simulink model "SSN_39busRT_Ctrl_4WT_19B"  (R2021a)
settings: Solver=ode3  StartTime=0.0  StopTime=10  FixedStep=Ts  MaxStep=1/60  RelTol=1e-2  AbsTol=1e-1
PreLoadFcn:
  | Ts=2.50e-6; ssn_ieee39_params; load('Pwf.mat');
InitFcn:
  | Ts=2.50e-6; ssn_ieee39_params; load('Pwf.mat');
values from neighbouring files (symbols this model uses):
  f = 50    [ssn_ieee39_params_ctrl.m]
  fNom = f    (= 60)    [ssn_ieee39_params_ctrl.m]
  ILR = 5.02    [ssn_ieee39_params_ctrl.m]
  IQMIN = 0.1    [ssn_ieee39_params_ctrl.m]
  ISCLIM = 1    [ssn_ieee39_params_ctrl.m]
  ITFpu = 1.10    (= 1.1)    [ssn_ieee39_params_ctrl.m]
  K = 1    [ssn_ieee39_params_ctrl.m]
  K1 = 1    [ssn_ieee39_params_ctrl.m]
  K2 = 2    [ssn_ieee39_params_ctrl.m]
  KCL = 1.04    [ssn_ieee39_params_ctrl.m]
  KFB = 0    [ssn_ieee39_params_ctrl.m]
  KFF = 1    [ssn_ieee39_params_ctrl.m]
  KFIX = 1    [ssn_ieee39_params_ctrl.m]
  KG = 1    [ssn_ieee39_params_ctrl.m]
  KIA = 59.91    [ssn_ieee39_params_ctrl.m]
  KIOEX = 0.0303    [ssn_ieee39_params_ctrl.m]
  KIUEX = 0.0303    [ssn_ieee39_params_ctrl.m]
  KIUOEX = 1    [ssn_ieee39_params_ctrl.m]
  KIUUEX = 1    [ssn_ieee39_params_ctrl.m]
  KLR = 22.47    [ssn_ieee39_params_ctrl.m]
  KM = 1    [ssn_ieee39_params_ctrl.m]
  KOEL = 0.24    [ssn_ieee39_params_ctrl.m]
  Kp = 1    [ssn_ieee39_params_ctrl.m]
  KPA = 30    [ssn_ieee39_params_ctrl.m]
  KPOEL = 1    [ssn_ieee39_params_ctrl.m]
  KPOEX = 0    [ssn_ieee39_params_ctrl.m]
  KPUEX = 0    [ssn_ieee39_params_ctrl.m]
  KSCALE = 0.319    [ssn_ieee39_params_ctrl.m]
  KUF = 0    [ssn_ieee39_params_ctrl.m]
  KUI = 0.001    [ssn_ieee39_params_ctrl.m]
  KUL = 0.24    [ssn_ieee39_params_ctrl.m]
  s = 10    [ssn_ieee39_params_ctrl.m]
  TA = 0.01    [ssn_ieee39_params_ctrl.m]
  Tadj = 0    [ssn_ieee39_params_ctrl.m]
  taps = [1 1 1.07 1.07 1.009 1.025 1 1.025 1.025 1.025]*1    [ssn_ieee39_params_ctrl.m]
  TF = 0.02    [ssn_ieee39_params_ctrl.m]
  TG = 0.024    [ssn_ieee39_params_ctrl.m]
  TINV = 0    [ssn_ieee39_params_ctrl.m]
  TIT = 0.1    [ssn_ieee39_params_ctrl.m]
  TL_10_11_len = 14    [ssn_ieee39_params_ctrl.m]
  TL_10_13_len = 14    [ssn_ieee39_params_ctrl.m]
  TL_13_14_len = 32    [ssn_ieee39_params_ctrl.m]
  TL_14_15_len = 70    [ssn_ieee39_params_ctrl.m]
  TL_15_16_len = 31.5    [ssn_ieee39_params_ctrl.m]
  TL_16_17_len = 26    [ssn_ieee39_params_ctrl.m]
  TL_16_19_len = 61    [ssn_ieee39_params_ctrl.m]
  TL_16_21_len = 46    [ssn_ieee39_params_ctrl.m]
  TL_16_24_len = 15    [ssn_ieee39_params_ctrl.m]
  TL_17_18_len = 26    [ssn_ieee39_params_ctrl.m]
  TL_17_27_len = 59    [ssn_ieee39_params_ctrl.m]
  TL_1_2_len = 134    [ssn_ieee39_params_ctrl.m]
  TL_1_39_len = 105    [ssn_ieee39_params_ctrl.m]
  TL_21_22_len = 47    [ssn_ieee39_params_ctrl.m]
  TL_22_23_len = 33    [ssn_ieee39_params_ctrl.m]
  TL_24_23_len = 88    [ssn_ieee39_params_ctrl.m]
  TL_25_26_len = 101    [ssn_ieee39_params_ctrl.m]
  TL_26_27_len = 46.5    [ssn_ieee39_params_ctrl.m]
  TL_26_28_len = 151    [ssn_ieee39_params_ctrl.m]
  TL_26_29_len = 200    [ssn_ieee39_params_ctrl.m]
  TL_28_29_len = 48    [ssn_ieee39_params_ctrl.m]
  TL_2_25_len = 28    [ssn_ieee39_params_ctrl.m]
  TL_2_2_len = 49    [ssn_ieee39_params_ctrl.m]
  TL_3_18_len = 42    [ssn_ieee39_params_ctrl.m]
  TL_3_4_len = 53    [ssn_ieee39_params_ctrl.m]
  TL_4_14_len = 33    [ssn_ieee39_params_ctrl.m]
  TL_4_5_len = 32.5    [ssn_ieee39_params_ctrl.m]
  TL_5_6_len = 14    [ssn_ieee39_params_ctrl.m]
  TL_5_8_len = 32    [ssn_ieee39_params_ctrl.m]
  TL_6_11_len = 26.5    [ssn_ieee39_params_ctrl.m]
  TL_6_7_len = 25.5    [ssn_ieee39_params_ctrl.m]
  TL_7_8_len = 15    [ssn_ieee39_params_ctrl.m]
  TL_8_9_len = 93    [ssn_ieee39_params_ctrl.m]
  TL_9_39_len = 136    [ssn_ieee39_params_ctrl.m]
  TOEL = 5.00    (= 5)    [ssn_ieee39_params_ctrl.m]
  TQREF = 0    [ssn_ieee39_params_ctrl.m]
  TQSCL = 0.012    [ssn_ieee39_params_ctrl.m]
  Ts_PMU = 1/1000    (= 0.001)    [ssn_ieee39_params_ctrl.m]
  TU1 = 0    [ssn_ieee39_params_ctrl.m]
  TU2 = 0    [ssn_ieee39_params_ctrl.m]
  TU3 = 0    [ssn_ieee39_params_ctrl.m]
  TU4 = 0    [ssn_ieee39_params_ctrl.m]
  TUL = 0    [ssn_ieee39_params_ctrl.m]
  TUP = 0.050    (= 0.05)    [ssn_ieee39_params_ctrl.m]
  TUQ = .005    (= 0.005)    [ssn_ieee39_params_ctrl.m]
  TUV = 0.2    [ssn_ieee39_params_ctrl.m]
  VAAMAX = VAMAX    (= 7.05)    [ssn_ieee39_params_ctrl.m]
  VAMAX = 7.05    [ssn_ieee39_params_ctrl.m]
  VAMIN = -6.11    [ssn_ieee39_params_ctrl.m]
  VBMAX = 999    [ssn_ieee39_params_ctrl.m]
  VF = 0    [ssn_ieee39_params_ctrl.m]
  VFB = 0    [ssn_ieee39_params_ctrl.m]
  VMMAX = 7.05    [ssn_ieee39_params_ctrl.m]
  VMMIN = -6.11    [ssn_ieee39_params_ctrl.m]
  VOELmax1 = 0.2353    [ssn_ieee39_params_ctrl.m]
  VOELmax2 = 0.0    (= 0)    [ssn_ieee39_params_ctrl.m]
  VOELmin1 = -0.24    [ssn_ieee39_params_ctrl.m]
  VOELmin2 = -1.0    (= -1)    [ssn_ieee39_params_ctrl.m]
  VRMAX = 7.05    [ssn_ieee39_params_ctrl.m]
  VRMIN = -6.11    [ssn_ieee39_params_ctrl.m]
  VSCLmax = 0.20    (= 0.2)    [ssn_ieee39_params_ctrl.m]
  VSCLmin = -0.10    (= -0.1)    [ssn_ieee39_params_ctrl.m]
  VUELmax1 = 1    [ssn_ieee39_params_ctrl.m]
  VUELmax2 = 1    [ssn_ieee39_params_ctrl.m]
  VUELmin1 = -1    [ssn_ieee39_params_ctrl.m]
  VUELmin2 = -1    [ssn_ieee39_params_ctrl.m]
  VUImax = 1    [ssn_ieee39_params_ctrl.m]
  VUImin = -1    [ssn_ieee39_params_ctrl.m]
undefined symbols (not defined in the file or in its folder): another_event_name, D1, Delta, DiscIntNeverNeededParam, find_system, MOV_segment9, my_event_name, powergui, Pw1, Pw2, Pw3, Pw4, vNomHV
libraries: powerlib_extras x162, spsThreePhaseVIMeasurementLib x55, spsCurrentMeasurementLib x52, simulink_extras x44, slpidlib x40, op_dpl_lib x36, spsST2AModel x20, spsThreePhaseParallelRLCLoadLib x20, spsThreePhaseTransformerTwoWindingsLib x17, spsControlledVoltageSourceLib x16, spsVoltageMeasurementLib x12, spsSynchronousMachinepuStandardLib x10
(part 5 of 19)

== system SSN_39busRT_Ctrl_4WT_19B/SM_master/G10/G10 ==
  note: Rotor Speed
  note: Rotor Speed Reference
  note: SM Measurement Signal
  note: Active Power
  note: Field Current
  note: Voltage Reference
  note: Stator Voltage
  note: Reactive Power
  note: Stator Current
  note: Field Voltage (Vf)
  note: Mechanical
      | Power (Pm)
  note: Measurement Outputs
  note: Rotor Speed
  note: Active Power
  note: Stator Voltage
  note: Stator Current
  note: Field Current
  note: Reactive Power
  wref (pu) : Inport
  Vref (pu) : Inport  Port=2
  "Generator Measurements " : Subsystem
  "Governor model " : Subsystem
  Ground7 : Ground
  ST6C EXCITER-1 : Subsystem
  Synchronous Machine : spsSynchronousMachinepuStandardLib/Synchronous Machine pu Standard  PresetModel=No  MechanicalLoad=Mechanical power Pm  ShowDetailedParameters=on  RotorType=Salient-pole  Units=per unit standard parameters  MeasurementBus=off  NominalParameters="[ Pn  Vn   f ]"  Reactances1=[ 31 32 33 34 35 36 37 ]  Reactances2=[ 1.305, 0.296, 0.252, 0.474, 0.243, 0.18 ]  dAxisTimeConstants=Short-circuit  qAxisTimeConstants=Open-circuit  TimeConstants1=[]  TimeConstants2=[]  TimeConstants3=[]  TimeConstants4=[]  TimeConstants5=[ 1.01, 0.053, 0.1 ]  TimeConstants6=[]  TimeConstants7=[]  TimeConstants8=[]  StatorResistance=2.8544e-3  Mechanical=[H1 0 2]  PolePairs=2  InitialConditions=[0 -62.5202 1.01055 1.01055 1.01055 8.25986 -111.74 128.26 1.32748]  SetSaturation=off  Saturation=[0.6404,0.7127,0.8441,0.9214,0.9956,1.082,1.19,1.316,1.457;0.7,0.7698,0.8872,0.9466,0.9969,1.046,1.1,1.151,1.201]  LoadFlowParameters=[1 150000000 0 0]  TsPowergui=0  TsBlock=-1  IterativeModel=Trapezoidal non iterative  IterativeDiscreteModel=Trapezoidal non iterative  BusType=PV  Pref=42e6  Qref=0  Qmin=-50000000  Qmax=50000000  PLF=0  QLF=0
      settings: SourceProductBaseCode=PS
  A : PMIOPort  Side=Right
  B : PMIOPort  Port=2  Side=Right
  C : PMIOPort  Port=3  Side=Right
  sm1 : Outport  VectorParamsAs1DForOutWhenUnconnected=off
  wires:
  [PT1st] -> "Governor model "/3(Input)
  [Ifd1st] -> ST6C EXCITER-1/4(Ifd)
  [Vt1st] -> ST6C EXCITER-1/2(Vt)
  [wm1] -> "Governor model "/2(w (pu))
  "Generator Measurements "/3(Vt) -> [Vt1st]
  "Generator Measurements "/6(PT) -> [PT1st]
  "Generator Measurements "/7(QT) -> [QT1st]
  "Generator Measurements "/1(sm) -> sm1/1
  "Generator Measurements "/5(It) -> [It1st]
  "Generator Measurements "/4(Ifd) -> [Ifd1st]
  "Generator Measurements "/2(wm) -> [wm1]
  ST6C EXCITER-1/1(Efd) -> Synchronous Machine/2, [Efd1st]
  [PT1st] -> ST6C EXCITER-1/7(PT)
  [It1st] -> ST6C EXCITER-1/3(It)
  [QT1st] -> ST6C EXCITER-1/6(QT)
  Ground7/1 -> ST6C EXCITER-1/5(Vstab)
  wref (pu)/1 -> "Governor model "/1(wref (pu)1)
  "Governor model "/1(Pmec (pu)) -> Synchronous Machine/1
  Vref (pu)/1 -> ST6C EXCITER-1/1(Vref)
  Synchronous Machine/1 -> "Generator Measurements "/1(m)
  connections:
  A/RConn1 -- Synchronous Machine/RConn1
  C/RConn1 -- Synchronous Machine/RConn3
  B/RConn1 -- Synchronous Machine/RConn2

== system SSN_39busRT_Ctrl_4WT_19B/SM_master/G2/G2 ==
  note: Reactive Power
  note: Field Current
  note: Stator Current
  note: Stator Voltage
  note: Active Power
  note: Rotor Speed
  note: Measurement Outputs
  note: Mechanical
      | Power (Pm)
  note: Field Voltage (Vf)
  note: Stator Current
  note: Reactive Power
  note: Stator Voltage
  note: Voltage Reference
  note: Field Current
  note: Active Power
  note: SM Measurement Signal
  note: Rotor Speed Reference
  note: Rotor Speed
  wref (pu) : Inport
  Vref (pu) : Inport  Port=2
  Generator Measurements (Output) : Subsystem
  "Governor model " : Subsystem
  Ground7 : Ground
  ST6C EXCITER-1 : Subsystem
  Synchronous Machine : spsSynchronousMachinepuStandardLib/Synchronous Machine pu Standard  PresetModel=No  MechanicalLoad=Mechanical power Pm  ShowDetailedParameters=on  RotorType=Salient-pole  Units=per unit standard parameters  MeasurementBus=off  NominalParameters="[ Pn  Vn   f ]"  Reactances1=[ 31 32 33 34 35 36 37 ]  Reactances2=[ 1.305, 0.296, 0.252, 0.474, 0.243, 0.18 ]  dAxisTimeConstants=Short-circuit  qAxisTimeConstants=Open-circuit  TimeConstants1=[]  TimeConstants2=[]  TimeConstants3=[]  TimeConstants4=[]  TimeConstants5=[ 1.01, 0.053, 0.1 ]  TimeConstants6=[]  TimeConstants7=[]  TimeConstants8=[]  StatorResistance=2.8544e-3  Mechanical=[H1 0 2]  PolePairs=2  InitialConditions=[0 -62.5202 1.01055 1.01055 1.01055 8.25986 -111.74 128.26 1.32748]  SetSaturation=off  Saturation=[0.6404,0.7127,0.8441,0.9214,0.9956,1.082,1.19,1.316,1.457;0.7,0.7698,0.8872,0.9466,0.9969,1.046,1.1,1.151,1.201]  LoadFlowParameters=[1 150000000 0 0]  TsPowergui=0  TsBlock=-1  IterativeModel=Trapezoidal non iterative  IterativeDiscreteModel=Trapezoidal non iterative  BusType=PV  Pref=42e6  Qref=0  Qmin=-50000000  Qmax=50000000  PLF=0  QLF=0
      settings: SourceProductBaseCode=PS
  A : PMIOPort  Side=Right
  B : PMIOPort  Port=2  Side=Right
  C : PMIOPort  Port=3  Side=Right
  sm1 : Outport  VectorParamsAs1DForOutWhenUnconnected=off
  wires:
  Synchronous Machine/1 -> Generator Measurements (Output)/1(m)
  Vref (pu)/1 -> ST6C EXCITER-1/1(Vref)
  "Governor model "/1(Pmec (pu)) -> Synchronous Machine/1
  wref (pu)/1 -> "Governor model "/1(wref (pu)1)
  Ground7/1 -> ST6C EXCITER-1/5(Vstab)
  [QT1st] -> ST6C EXCITER-1/6(QT)
  [It1st] -> ST6C EXCITER-1/3(It)
  [PT1st] -> ST6C EXCITER-1/7(PT)
  ST6C EXCITER-1/1(Efd) -> [Efd1st], Synchronous Machine/2
  Generator Measurements (Output)/2(wm) -> [wm1]
  Generator Measurements (Output)/4(Ifd) -> [Ifd1st]
  Generator Measurements (Output)/5(It) -> [It1st]
  Generator Measurements (Output)/1(sm) -> sm1/1
  Generator Measurements (Output)/7(QT) -> [QT1st]
  Generator Measurements (Output)/6(PT) -> [PT1st]
  Generator Measurements (Output)/3(Vt) -> [Vt1st]
  [wm1] -> "Governor model "/2(w (pu))
  [Vt1st] -> ST6C EXCITER-1/2(Vt)
  [Ifd1st] -> ST6C EXCITER-1/4(Ifd)
  [PT1st] -> "Governor model "/3(Input)
  connections:
  B/RConn1 -- Synchronous Machine/RConn2
  C/RConn1 -- Synchronous Machine/RConn3
  A/RConn1 -- Synchronous Machine/RConn1

== system SSN_39busRT_Ctrl_4WT_19B/SM_master/G3/G3 ==
  note: Rotor Speed
  note: Rotor Speed Reference
  note: SM Measurement Signal
  note: Active Power
  note: Field Current
  note: Voltage Reference
  note: Stator Voltage
  note: Reactive Power
  note: Stator Current
  note: Field Voltage (Vf)
  note: Synchronous
      | Machine
      | - Phase A
      | - Phase B
      | - Phase C
  note: Mechanical
      | Power (Pm)
  note: Selected (Combined)
      | Synchronous Machine
      | Measurement Outputs
  note: Rotor Speed
  note: Active Power
  note: Stator Voltage
  note: Stator Current
  note: Field Current
  note: Reactive Power
  wref (pu) : Inport
  Vref (pu) : Inport  Port=2
  Generator Measurements (Output) : Subsystem
  Governor model with Droop : Subsystem
  Ground7 : Ground
  ST6C EXCITER-1 : Subsystem
  Synchronous Machine : spsSynchronousMachinepuStandardLib/Synchronous Machine pu Standard  PresetModel=No  MechanicalLoad=Mechanical power Pm  ShowDetailedParameters=on  RotorType=Salient-pole  Units=per unit standard parameters  MeasurementBus=off  NominalParameters="[ Pn  Vn   f ]"  Reactances1=[ 31 32 33 34 35 36 37 ]  Reactances2=[ 1.305, 0.296, 0.252, 0.474, 0.243, 0.18 ]  dAxisTimeConstants=Short-circuit  qAxisTimeConstants=Open-circuit  TimeConstants1=[]  TimeConstants2=[]  TimeConstants3=[]  TimeConstants4=[]  TimeConstants5=[ 1.01, 0.053, 0.1 ]  TimeConstants6=[]  TimeConstants7=[]  TimeConstants8=[]  StatorResistance=2.8544e-3  Mechanical=[H1 0 2]  PolePairs=2  InitialConditions=[0 -62.5202 1.01055 1.01055 1.01055 8.25986 -111.74 128.26 1.32748]  SetSaturation=off  Saturation=[0.6404,0.7127,0.8441,0.9214,0.9956,1.082,1.19,1.316,1.457;0.7,0.7698,0.8872,0.9466,0.9969,1.046,1.1,1.151,1.201]  LoadFlowParameters=[1 150000000 0 0]  TsPowergui=0  TsBlock=-1  IterativeModel=Trapezoidal non iterative  IterativeDiscreteModel=Trapezoidal non iterative  BusType=PV  Pref=42e6  Qref=0  Qmin=-50000000  Qmax=50000000  PLF=0  QLF=0
      settings: SourceProductBaseCode=PS
  A : PMIOPort  Side=Right
  B : PMIOPort  Port=2  Side=Right
  C : PMIOPort  Port=3  Side=Right
  sm1 : Outport  VectorParamsAs1DForOutWhenUnconnected=off
  wires:
  [PT1st] -> Governor model with Droop/3(Input)
  [Ifd1st] -> ST6C EXCITER-1/4(Ifd)
  [Vt1st] -> ST6C EXCITER-1/2(Vt)
  [wm1] -> Governor model with Droop/2(w (pu))
  Generator Measurements (Output)/3(Vt) -> [Vt1st]
  Generator Measurements (Output)/6(PT) -> [PT1st]
  Generator Measurements (Output)/7(QT) -> [QT1st]
  Generator Measurements (Output)/1(sm) -> sm1/1
  Generator Measurements (Output)/5(It) -> [It1st]
  Generator Measurements (Output)/4(Ifd) -> [Ifd1st]
  Generator Measurements (Output)/2(wm) -> [wm1]
  ST6C EXCITER-1/1(Efd) -> Synchronous Machine/2, [Efd1st]
  [PT1st] -> ST6C EXCITER-1/7(PT)
  [It1st] -> ST6C EXCITER-1/3(It)
  [QT1st] -> ST6C EXCITER-1/6(QT)
  Ground7/1 -> ST6C EXCITER-1/5(Vstab)
  wref (pu)/1 -> Governor model with Droop/1(wref (pu)1)
  Governor model with Droop/1(Pmec (pu)) -> Synchronous Machine/1
  Vref (pu)/1 -> ST6C EXCITER-1/1(Vref)
  Synchronous Machine/1 -> Generator Measurements (Output)/1(m)
  connections:
  A/RConn1 -- Synchronous Machine/RConn1
  C/RConn1 -- Synchronous Machine/RConn3
  B/RConn1 -- Synchronous Machine/RConn2

== system SSN_39busRT_Ctrl_4WT_19B/SM_master/G4/G4 ==
  note: Rotor Speed
  note: Rotor Speed Reference
  note: SM Measurement Signal
  note: Active Power
  note: Field Current
  note: Voltage Reference
  note: Stator Voltage
  note: Reactive Power
  note: Stator Current
  note: Field Voltage (Vf)
  note: Mechanical
      | Power (Pm)
  note: Measurement Outputs
  note: Rotor Speed
  note: Active Power
  note: Stator Voltage
  note: Stator Current
  note: Field Current
  note: Reactive Power
  wref (pu) : Inport
  Vref (pu) : Inport  Port=2
  Generator Measurements (Output) : Subsystem
  "Governor model " : Subsystem
  Ground7 : Ground
  ST6C EXCITER-1 : Subsystem
  Synchronous Machine : spsSynchronousMachinepuStandardLib/Synchronous Machine pu Standard  PresetModel=No  MechanicalLoad=Mechanical power Pm  ShowDetailedParameters=on  RotorType=Salient-pole  Units=per unit standard parameters  MeasurementBus=off  NominalParameters="[ Pn  Vn   f ]"  Reactances1=[ 31 32 33 34 35 36 37 ]  Reactances2=[ 1.305, 0.296, 0.252, 0.474, 0.243, 0.18 ]  dAxisTimeConstants=Short-circuit  qAxisTimeConstants=Open-circuit  TimeConstants1=[]  TimeConstants2=[]  TimeConstants3=[]  TimeConstants4=[]  TimeConstants5=[ 1.01, 0.053, 0.1 ]  TimeConstants6=[]  TimeConstants7=[]  TimeConstants8=[]  StatorResistance=2.8544e-3  Mechanical=[H1 0 2]  PolePairs=2  InitialConditions=[0 -62.5202 1.01055 1.01055 1.01055 8.25986 -111.74 128.26 1.32748]  SetSaturation=off  Saturation=[0.6404,0.7127,0.8441,0.9214,0.9956,1.082,1.19,1.316,1.457;0.7,0.7698,0.8872,0.9466,0.9969,1.046,1.1,1.151,1.201]  LoadFlowParameters=[1 150000000 0 0]  TsPowergui=0  TsBlock=-1  IterativeModel=Trapezoidal non iterative  IterativeDiscreteModel=Trapezoidal non iterative  BusType=PV  Pref=42e6  Qref=0  Qmin=-50000000  Qmax=50000000  PLF=0  QLF=0
      settings: SourceProductBaseCode=PS
  A : PMIOPort  Side=Right
  B : PMIOPort  Port=2  Side=Right
  C : PMIOPort  Port=3  Side=Right
  sm1 : Outport  VectorParamsAs1DForOutWhenUnconnected=off
  wires:
  [PT1st] -> "Governor model "/3(Input)
  [Ifd1st] -> ST6C EXCITER-1/4(Ifd)
  [Vt1st] -> ST6C EXCITER-1/2(Vt)
  [wm1] -> "Governor model "/2(w (pu))
  Generator Measurements (Output)/3(Vt) -> [Vt1st]
  Generator Measurements (Output)/6(PT) -> [PT1st]
  Generator Measurements (Output)/7(QT) -> [QT1st]
  Generator Measurements (Output)/1(sm) -> sm1/1
  Generator Measurements (Output)/5(It) -> [It1st]
  Generator Measurements (Output)/4(Ifd) -> [Ifd1st]
  Generator Measurements (Output)/2(wm) -> [wm1]
  ST6C EXCITER-1/1(Efd) -> Synchronous Machine/2, [Efd1st]
  [PT1st] -> ST6C EXCITER-1/7(PT)
  [It1st] -> ST6C EXCITER-1/3(It)
  [QT1st] -> ST6C EXCITER-1/6(QT)
  Ground7/1 -> ST6C EXCITER-1/5(Vstab)
  wref (pu)/1 -> "Governor model "/1(wref (pu)1)
  "Governor model "/1(Pmec (pu)) -> Synchronous Machine/1
  Vref (pu)/1 -> ST6C EXCITER-1/1(Vref)
  Synchronous Machine/1 -> Generator Measurements (Output)/1(m)
  connections:
  A/RConn1 -- Synchronous Machine/RConn1
  C/RConn1 -- Synchronous Machine/RConn3
  B/RConn1 -- Synchronous Machine/RConn2

== system SSN_39busRT_Ctrl_4WT_19B/SM_master/G5/G5 ==
  note: Reactive Power
  note: Field Current
  note: Stator Current
  note: Stator Voltage
  note: Active Power
  note: Rotor Speed
  note: Selected (Combined)
      | Synchronous Machine
      | Measurement Outputs
  note: Mechanical
      | Power (Pm)
  note: Synchronous
      | Machine
      | - Phase A
      | - Phase B
      | - Phase C
  note: Field Voltage (Vf)
  note: Stator Current
  note: Reactive Power
  note: Stator Voltage
  note: Voltage Reference
  note: Field Current
  note: Active Power
  note: SM Measurement Signal
  note: Rotor Speed Reference
  note: Rotor Speed
  wref (pu) : Inport
  Vref (pu) : Inport  Port=2
  Generator Measurements (Output) : Subsystem
  Governor model with Droop : Subsystem
  Ground7 : Ground
  ST6C EXCITER-1 : Subsystem
  Synchronous Machine : spsSynchronousMachinepuStandardLib/Synchronous Machine pu Standard  PresetModel=No  MechanicalLoad=Mechanical power Pm  ShowDetailedParameters=on  RotorType=Salient-pole  Units=per unit standard parameters  MeasurementBus=off  NominalParameters="[ Pn  Vn   f ]"  Reactances1=[ 31 32 33 34 35 36 37 ]  Reactances2=[ 1.305, 0.296, 0.252, 0.474, 0.243, 0.18 ]  dAxisTimeConstants=Short-circuit  qAxisTimeConstants=Open-circuit  TimeConstants1=[]  TimeConstants2=[]  TimeConstants3=[]  TimeConstants4=[]  TimeConstants5=[ 1.01, 0.053, 0.1 ]  TimeConstants6=[]  TimeConstants7=[]  TimeConstants8=[]  StatorResistance=2.8544e-3  Mechanical=[H1 0 2]  PolePairs=2  InitialConditions=[0 -62.5202 1.01055 1.01055 1.01055 8.25986 -111.74 128.26 1.32748]  SetSaturation=off  Saturation=[0.6404,0.7127,0.8441,0.9214,0.9956,1.082,1.19,1.316,1.457;0.7,0.7698,0.8872,0.9466,0.9969,1.046,1.1,1.151,1.201]  LoadFlowParameters=[1 150000000 0 0]  TsPowergui=0  TsBlock=-1  IterativeModel=Trapezoidal non iterative  IterativeDiscreteModel=Trapezoidal non iterative  BusType=PV  Pref=42e6  Qref=0  Qmin=-50000000  Qmax=50000000  PLF=0  QLF=0
      settings: SourceProductBaseCode=PS
  A : PMIOPort  Side=Right
  B : PMIOPort  Port=2  Side=Right
  C : PMIOPort  Port=3  Side=Right
  sm1 : Outport  VectorParamsAs1DForOutWhenUnconnected=off
  wires:
  Synchronous Machine/1 -> Generator Measurements (Output)/1(m)
  Vref (pu)/1 -> ST6C EXCITER-1/1(Vref)
  Governor model with Droop/1(Pmec (pu)) -> Synchronous Machine/1
  wref (pu)/1 -> Governor model with Droop/1(wref (pu)1)
  Ground7/1 -> ST6C EXCITER-1/5(Vstab)
  [QT1st] -> ST6C EXCITER-1/6(QT)
  [It1st] -> ST6C EXCITER-1/3(It)
  [PT1st] -> ST6C EXCITER-1/7(PT)
  ST6C EXCITER-1/1(Efd) -> [Efd1st], Synchronous Machine/2
  Generator Measurements (Output)/2(wm) -> [wm1]
  Generator Measurements (Output)/4(Ifd) -> [Ifd1st]
  Generator Measurements (Output)/5(It) -> [It1st]
  Generator Measurements (Output)/1(sm) -> sm1/1
  Generator Measurements (Output)/7(QT) -> [QT1st]
  Generator Measurements (Output)/6(PT) -> [PT1st]
  Generator Measurements (Output)/3(Vt) -> [Vt1st]
  [wm1] -> Governor model with Droop/2(w (pu))
  [Vt1st] -> ST6C EXCITER-1/2(Vt)
  [Ifd1st] -> ST6C EXCITER-1/4(Ifd)
  [PT1st] -> Governor model with Droop/3(Input)
  connections:
  B/RConn1 -- Synchronous Machine/RConn2
  C/RConn1 -- Synchronous Machine/RConn3
  A/RConn1 -- Synchronous Machine/RConn1

== system SSN_39busRT_Ctrl_4WT_19B/SM_master/G6/G6 ==
  note: Rotor Speed
  note: Rotor Speed Reference
  note: SM Measurement Signal
  note: Active Power
  note: Field Current
  note: Voltage Reference
  note: Stator Voltage
  note: Reactive Power
  note: Stator Current
  note: Field Voltage (Vf)
  note: Mechanical
      | Power (Pm)
  note: Measurement Outputs
  note: Rotor Speed
  note: Active Power
  note: Stator Voltage
  note: Stator Current
  note: Field Current
  note: Reactive Power
  wref (pu) : Inport
  Vref (pu) : Inport  Port=2
  Generator Measurements (Output) : Subsystem
  Governor model with Droop : Subsystem
  Ground7 : Ground
  ST6C EXCITER-1 : Subsystem
  Synchronous Machine : spsSynchronousMachinepuStandardLib/Synchronous Machine pu Standard  PresetModel=No  MechanicalLoad=Mechanical power Pm  ShowDetailedParameters=on  RotorType=Salient-pole  Units=per unit standard parameters  MeasurementBus=off  NominalParameters="[ Pn  Vn   f ]"  Reactances1=[ 31 32 33 34 35 36 37 ]  Reactances2=[ 1.305, 0.296, 0.252, 0.474, 0.243, 0.18 ]  dAxisTimeConstants=Short-circuit  qAxisTimeConstants=Open-circuit  TimeConstants1=[]  TimeConstants2=[]  TimeConstants3=[]  TimeConstants4=[]  TimeConstants5=[ 1.01, 0.053, 0.1 ]  TimeConstants6=[]  TimeConstants7=[]  TimeConstants8=[]  StatorResistance=2.8544e-3  Mechanical=[H1 0 2]  PolePairs=2  InitialConditions=[0 -62.5202 1.01055 1.01055 1.01055 8.25986 -111.74 128.26 1.32748]  SetSaturation=off  Saturation=[0.6404,0.7127,0.8441,0.9214,0.9956,1.082,1.19,1.316,1.457;0.7,0.7698,0.8872,0.9466,0.9969,1.046,1.1,1.151,1.201]  LoadFlowParameters=[1 150000000 0 0]  TsPowergui=0  TsBlock=-1  IterativeModel=Trapezoidal non iterative  IterativeDiscreteModel=Trapezoidal non iterative  BusType=PV  Pref=42e6  Qref=0  Qmin=-50000000  Qmax=50000000  PLF=0  QLF=0
      settings: SourceProductBaseCode=PS
  A : PMIOPort  Side=Right
  B : PMIOPort  Port=2  Side=Right
  C : PMIOPort  Port=3  Side=Right
  sm1 : Outport  VectorParamsAs1DForOutWhenUnconnected=off
  wires:
  [PT1st] -> Governor model with Droop/3(Input)
  [Ifd1st] -> ST6C EXCITER-1/4(Ifd)
  [Vt1st] -> ST6C EXCITER-1/2(Vt)
  [wm1] -> Governor model with Droop/2(w (pu))
  Generator Measurements (Output)/3(Vt) -> [Vt1st]
  Generator Measurements (Output)/6(PT) -> [PT1st]
  Generator Measurements (Output)/7(QT) -> [QT1st]
  Generator Measurements (Output)/1(sm) -> sm1/1
  Generator Measurements (Output)/5(It) -> [It1st]
  Generator Measurements (Output)/4(Ifd) -> [Ifd1st]
  Generator Measurements (Output)/2(wm) -> [wm1]
  ST6C EXCITER-1/1(Efd) -> Synchronous Machine/2, [Efd1st]
  [PT1st] -> ST6C EXCITER-1/7(PT)
  [It1st] -> ST6C EXCITER-1/3(It)
  [QT1st] -> ST6C EXCITER-1/6(QT)
  Ground7/1 -> ST6C EXCITER-1/5(Vstab)
  wref (pu)/1 -> Governor model with Droop/1(wref (pu)1)
  Governor model with Droop/1(Pmec (pu)) -> Synchronous Machine/1
  Vref (pu)/1 -> ST6C EXCITER-1/1(Vref)
  Synchronous Machine/1 -> Generator Measurements (Output)/1(m)
  connections:
  A/RConn1 -- Synchronous Machine/RConn1
  C/RConn1 -- Synchronous Machine/RConn3
  B/RConn1 -- Synchronous Machine/RConn2

== system SSN_39busRT_Ctrl_4WT_19B/SM_master/G7/G7 ==
  note: Rotor Speed
  note: Rotor Speed Reference
  note: SM Measurement Signal
  note: Active Power
  note: Field Current
  note: Voltage Reference
  note: Stator Voltage
  note: Reactive Power
  note: Stator Current
  note: Field Voltage (Vf)
  note: Mechanical
      | Power (Pm)
  note: Measurement Outputs
  note: Rotor Speed
  note: Active Power
  note: Stator Voltage
  note: Stator Current
  note: Field Current
  note: Reactive Power
  wref (pu) : Inport
  Vref (pu) : Inport  Port=2
  Generator Measurements (Output) : Subsystem
  Governor model with Droop : Subsystem
  Ground7 : Ground
  ST6C EXCITER-1 : Subsystem
  Synchronous Machine : spsSynchronousMachinepuStandardLib/Synchronous Machine pu Standard  PresetModel=No  MechanicalLoad=Mechanical power Pm  ShowDetailedParameters=on  RotorType=Salient-pole  Units=per unit standard parameters  MeasurementBus=off  NominalParameters="[ Pn  Vn   f ]"  Reactances1=[ 31 32 33 34 35 36 37 ]  Reactances2=[ 1.305, 0.296, 0.252, 0.474, 0.243, 0.18 ]  dAxisTimeConstants=Short-circuit  qAxisTimeConstants=Open-circuit  TimeConstants1=[]  TimeConstants2=[]  TimeConstants3=[]  TimeConstants4=[]  TimeConstants5=[ 1.01, 0.053, 0.1 ]  TimeConstants6=[]  TimeConstants7=[]  TimeConstants8=[]  StatorResistance=2.8544e-3  Mechanical=[H1 0 2]  PolePairs=2  InitialConditions=[0 -62.5202 1.01055 1.01055 1.01055 8.25986 -111.74 128.26 1.32748]  SetSaturation=off  Saturation=[0.6404,0.7127,0.8441,0.9214,0.9956,1.082,1.19,1.316,1.457;0.7,0.7698,0.8872,0.9466,0.9969,1.046,1.1,1.151,1.201]  LoadFlowParameters=[1 150000000 0 0]  TsPowergui=0  TsBlock=-1  IterativeModel=Trapezoidal non iterative  IterativeDiscreteModel=Trapezoidal non iterative  BusType=PV  Pref=42e6  Qref=0  Qmin=-50000000  Qmax=50000000  PLF=0  QLF=0
      settings: SourceProductBaseCode=PS
  A : PMIOPort  Side=Right
  B : PMIOPort  Port=2  Side=Right
  C : PMIOPort  Port=3  Side=Right
  sm1 : Outport  VectorParamsAs1DForOutWhenUnconnected=off
  wires:
  [PT1st] -> Governor model with Droop/3(Input)
  [Ifd1st] -> ST6C EXCITER-1/4(Ifd)
  [Vt1st] -> ST6C EXCITER-1/2(Vt)
  [wm1] -> Governor model with Droop/2(w (pu))
  Generator Measurements (Output)/3(Vt) -> [Vt1st]
  Generator Measurements (Output)/6(PT) -> [PT1st]
  Generator Measurements (Output)/7(QT) -> [QT1st]
  Generator Measurements (Output)/1(sm) -> sm1/1
  Generator Measurements (Output)/5(It) -> [It1st]
  Generator Measurements (Output)/4(Ifd) -> [Ifd1st]
  Generator Measurements (Output)/2(wm) -> [wm1]
  ST6C EXCITER-1/1(Efd) -> Synchronous Machine/2, [Efd1st]
  [PT1st] -> ST6C EXCITER-1/7(PT)
  [It1st] -> ST6C EXCITER-1/3(It)
  [QT1st] -> ST6C EXCITER-1/6(QT)
  Ground7/1 -> ST6C EXCITER-1/5(Vstab)
  wref (pu)/1 -> Governor model with Droop/1(wref (pu)1)
  Governor model with Droop/1(Pmec (pu)) -> Synchronous Machine/1
  Vref (pu)/1 -> ST6C EXCITER-1/1(Vref)
  Synchronous Machine/1 -> Generator Measurements (Output)/1(m)
  connections:
  A/RConn1 -- Synchronous Machine/RConn1
  C/RConn1 -- Synchronous Machine/RConn3
  B/RConn1 -- Synchronous Machine/RConn2

== system SSN_39busRT_Ctrl_4WT_19B/SM_master/G8/ G8 ==
  note: Reactive Power
  note: Field Current
  note: Stator Current
  note: Stator Voltage
  note: Active Power
  note: Rotor Speed
  note: Measurement Outputs
  note: Mechanical
      | Power (PU)
  note: Field Voltage (Vf PU)
  note: Stator Current
  note: Reactive Power
  note: Stator Voltage
  note: Voltage Reference
  note: Field Current
  note: Active Power
  note: SM Measurement Signal
  note: Rotor Speed Reference
  note: Rotor Speed
  wref (pu) : Inport
  Vref (pu) : Inport  Port=2
  "Generator Measurements " : Subsystem
  "Governor model " : Subsystem
  Ground7 : Ground
  ST6C EXCITER-1 : Subsystem
  Synchronous Machine : spsSynchronousMachinepuStandardLib/Synchronous Machine pu Standard  PresetModel=No  MechanicalLoad=Mechanical power Pm  ShowDetailedParameters=on  RotorType=Salient-pole  Units=per unit standard parameters  MeasurementBus=off  NominalParameters="[ Pn  Vn   f ]"  Reactances1=[ 31 32 33 34 35 36 37 ]  Reactances2=[ 1.305, 0.296, 0.252, 0.474, 0.243, 0.18 ]  dAxisTimeConstants=Short-circuit  qAxisTimeConstants=Open-circuit  TimeConstants1=[]  TimeConstants2=[]  TimeConstants3=[]  TimeConstants4=[]  TimeConstants5=[ 1.01, 0.053, 0.1 ]  TimeConstants6=[]  TimeConstants7=[]  TimeConstants8=[]  StatorResistance=2.8544e-3  Mechanical=[H1 0 2]  PolePairs=2  InitialConditions=[0 -62.5202 1.01055 1.01055 1.01055 8.25986 -111.74 128.26 1.32748]  SetSaturation=off  Saturation=[0.6404,0.7127,0.8441,0.9214,0.9956,1.082,1.19,1.316,1.457;0.7,0.7698,0.8872,0.9466,0.9969,1.046,1.1,1.151,1.201]  LoadFlowParameters=[1 150000000 0 0]  TsPowergui=0  TsBlock=-1  IterativeModel=Trapezoidal non iterative  IterativeDiscreteModel=Trapezoidal non iterative  BusType=PV  Pref=42e6  Qref=0  Qmin=-50000000  Qmax=50000000  PLF=0  QLF=0
      settings: SourceProductBaseCode=PS
  A : PMIOPort  Side=Right
  B : PMIOPort  Port=2  Side=Right
  C : PMIOPort  Port=3  Side=Right
  sm1 : Outport  VectorParamsAs1DForOutWhenUnconnected=off
  wires:
  Synchronous Machine/1 -> "Generator Measurements "/1(m)
  Vref (pu)/1 -> ST6C EXCITER-1/1(Vref)
  "Governor model "/1(Pmec (pu)) -> Synchronous Machine/1
  wref (pu)/1 -> "Governor model "/1(wref (pu)1)
  Ground7/1 -> ST6C EXCITER-1/5(Vstab)
  [QT1st] -> ST6C EXCITER-1/6(QT)
  [It1st] -> ST6C EXCITER-1/3(It)
  [PT1st] -> ST6C EXCITER-1/7(PT)
  ST6C EXCITER-1/1(Efd) -> [Efd1st], Synchronous Machine/2
  "Generator Measurements "/2(wm) -> [wm1]
  "Generator Measurements "/4(Ifd) -> [Ifd1st]
  "Generator Measurements "/5(It) -> [It1st]
  "Generator Measurements "/1(sm) -> sm1/1
  "Generator Measurements "/7(QT) -> [QT1st]
  "Generator Measurements "/6(PT) -> [PT1st]
  "Generator Measurements "/3(Vt) -> [Vt1st]
  [wm1] -> "Governor model "/2(w (pu))
  [Vt1st] -> ST6C EXCITER-1/2(Vt)
  [Ifd1st] -> ST6C EXCITER-1/4(Ifd)
  [PT1st] -> "Governor model "/3(Input)
  connections:
  B/RConn1 -- Synchronous Machine/RConn2
  C/RConn1 -- Synchronous Machine/RConn3
  A/RConn1 -- Synchronous Machine/RConn1

== system SSN_39busRT_Ctrl_4WT_19B/SM_master/G9/G9 ==
  note: Rotor Speed
  note: Rotor Speed Reference
  note: SM Measurement Signal
  note: Active Power
  note: Field Current
  note: Voltage Reference
  note: Stator Voltage
  note: Reactive Power
  note: Stator Current
  note: Field Voltage (Vf)
  note: Mechanical
      | Power (Pm)
  note: Measurement Outputs
  note: Rotor Speed
  note: Active Power
  note: Stator Voltage
  note: Stator Current
  note: Field Current
  note: Reactive Power
  wref (pu) : Inport
  Vref (pu) : Inport  Port=2
  Generator Measurements (Output) : Subsystem
  Governor model with Droop : Subsystem
  Ground7 : Ground
  ST6C EXCITER-1 : Subsystem
  Synchronous Machine : spsSynchronousMachinepuStandardLib/Synchronous Machine pu Standard  PresetModel=No  MechanicalLoad=Mechanical power Pm  ShowDetailedParameters=on  RotorType=Salient-pole  Units=per unit standard parameters  MeasurementBus=off  NominalParameters="[ Pn  Vn   f ]"  Reactances1=[ 31 32 33 34 35 36 37 ]  Reactances2=[ 1.305, 0.296, 0.252, 0.474, 0.243, 0.18 ]  dAxisTimeConstants=Short-circuit  qAxisTimeConstants=Open-circuit  TimeConstants1=[]  TimeConstants2=[]  TimeConstants3=[]  TimeConstants4=[]  TimeConstants5=[ 1.01, 0.053, 0.1 ]  TimeConstants6=[]  TimeConstants7=[]  TimeConstants8=[]  StatorResistance=2.8544e-3  Mechanical=[H1 0 2]  PolePairs=2  InitialConditions=[0 -62.5202 1.01055 1.01055 1.01055 8.25986 -111.74 128.26 1.32748]  SetSaturation=off  Saturation=[0.6404,0.7127,0.8441,0.9214,0.9956,1.082,1.19,1.316,1.457;0.7,0.7698,0.8872,0.9466,0.9969,1.046,1.1,1.151,1.201]  LoadFlowParameters=[1 150000000 0 0]  TsPowergui=0  TsBlock=-1  IterativeModel=Trapezoidal non iterative  IterativeDiscreteModel=Trapezoidal non iterative  BusType=PV  Pref=42e6  Qref=0  Qmin=-50000000  Qmax=50000000  PLF=0  QLF=0
      settings: SourceProductBaseCode=PS
  A : PMIOPort  Side=Right
  B : PMIOPort  Port=2  Side=Right
  C : PMIOPort  Port=3  Side=Right
  sm1 : Outport  VectorParamsAs1DForOutWhenUnconnected=off
  wires:
  [PT1st] -> Governor model with Droop/3(Input)
  [Ifd1st] -> ST6C EXCITER-1/4(Ifd)
  [Vt1st] -> ST6C EXCITER-1/2(Vt)
  [wm1] -> Governor model with Droop/2(w (pu))
  Generator Measurements (Output)/3(Vt) -> [Vt1st]
  Generator Measurements (Output)/6(PT) -> [PT1st]
  Generator Measurements (Output)/7(QT) -> [QT1st]
  Generator Measurements (Output)/1(sm) -> sm1/1
  Generator Measurements (Output)/5(It) -> [It1st]
  Generator Measurements (Output)/4(Ifd) -> [Ifd1st]
  Generator Measurements (Output)/2(wm) -> [wm1]
  ST6C EXCITER-1/1(Efd) -> Synchronous Machine/2, [Efd1st]
  [PT1st] -> ST6C EXCITER-1/7(PT)
  [It1st] -> ST6C EXCITER-1/3(It)
  [QT1st] -> ST6C EXCITER-1/6(QT)
  Ground7/1 -> ST6C EXCITER-1/5(Vstab)
  wref (pu)/1 -> Governor model with Droop/1(wref (pu)1)
  Governor model with Droop/1(Pmec (pu)) -> Synchronous Machine/1
  Vref (pu)/1 -> ST6C EXCITER-1/1(Vref)
  Synchronous Machine/1 -> Generator Measurements (Output)/1(m)
  connections:
  A/RConn1 -- Synchronous Machine/RConn1
  C/RConn1 -- Synchronous Machine/RConn3
  B/RConn1 -- Synchronous Machine/RConn2

== system SSN_39busRT_Ctrl_4WT_19B/powergui/EquivalentModel1/Sources ==
  Mux : Mux  Inputs=[1 1]
  u : Outport  VectorParamsAs1DForOutWhenUnconnected=off
  wires:
  Mux/1 -> u/1
  [T159_13809_39445529444035] -> Mux/1
  [T160_13858_39325123805635] -> Mux/2

== system SSN_39busRT_Ctrl_4WT_19B/powergui/EquivalentModel1/Yout ==
  v,i : Inport
  Demux : Demux  Outputs=[1 1 1]
  tag scope: T149_12942_36324237428855=global, T166_14587_45637003886935=global, T167_14636_45637984399065=global
  wires:
  v,i/1 -> Demux/1
  Demux/1 -> [T166_14587_45637003886935]
  Demux/2 -> [T167_14636_45637984399065]
  Demux/3 -> [T149_12942_36324237428855]

== system SSN_39busRT_Ctrl_4WT_19B/powergui/EquivalentModel10/Sources ==
  Mux : Mux  Inputs=[2 1 1 1 1 1 1 1 1 1 1 1 1]
  u : Outport  VectorParamsAs1DForOutWhenUnconnected=off
  wires:
  Mux/1 -> u/1
  [T67_5835_7808160989715] -> Mux/1
  [T74_6142_7947224238180] -> Mux/2
  [T74_6143_7948232813167] -> Mux/3
  [T74_6144_7949457397884] -> Mux/4
  [T75_6197_8147459697777] -> Mux/5
  [T75_6198_8148543724566] -> Mux/6
  [T75_6199_8149847124422] -> Mux/7
  [T74_6144_7943290167466] -> Mux/8
  [T74_6145_7944295233974] -> Mux/9
  [T74_6146_7945516310213] -> Mux/10
  [T75_6194_8151564869885] -> Mux/11
  [T75_6195_8152655070811] -> Mux/12
  [T75_6196_8153964644804] -> Mux/13

== system SSN_39busRT_Ctrl_4WT_19B/powergui/EquivalentModel10/Yout ==
  v,i : Inport
  Demux : Demux  Outputs=[2 1 1 1 1 1 1 1 1 1 1 1 1 1 1 1 1 1 1 1 1 1]
  tag scope: T55_4651_4630008375037=global, T55_4652_4632097164155=global, T55_4653_4634320376545=global, T55_4680_4617324042007=global, T55_4681_4619025875838=global, T55_4682_4621293204613=global, T56_4729_4742605101425=global, T56_4730_4744448642221=global, T56_4731_4746862521974=global, T67_5830_7741219315314=global, T77_6500_9525923614040=global, T77_6501_9526356872379=global, T77_6502_9521323067560=global, T77_6502_9527003805783=global, T77_6503_9521753040116=global, T77_6504_9522396687738=global, T78_6552_9766815931017=global, T78_6553_9767326097517=global, T78_6554_9768053289659=global, T78_6555_9761420549411=global, T78_6556_9761924928765=global, T78_6557_9762646333760=global
  wires:
  v,i/1 -> Demux/1
  Demux/1 -> [T67_5830_7741219315314]
  Demux/2 -> [T55_4680_4617324042007]
  Demux/3 -> [T55_4682_4621293204613]
  Demux/4 -> [T55_4681_4619025875838]
  Demux/5 -> [T56_4729_4742605101425]
  Demux/6 -> [T56_4731_4746862521974]
  Demux/7 -> [T56_4730_4744448642221]
  Demux/8 -> [T77_6500_9525923614040]
  Demux/9 -> [T77_6501_9526356872379]
  Demux/10 -> [T77_6502_9527003805783]
  Demux/11 -> [T78_6555_9761420549411]
  Demux/12 -> [T78_6556_9761924928765]
  Demux/13 -> [T78_6557_9762646333760]
  Demux/14 -> [T77_6502_9521323067560]
  Demux/15 -> [T77_6503_9521753040116]
  Demux/16 -> [T77_6504_9522396687738]
  Demux/17 -> [T78_6552_9766815931017]
  Demux/18 -> [T78_6553_9767326097517]
  Demux/19 -> [T78_6554_9768053289659]
  Demux/20 -> [T55_4651_4630008375037]
  Demux/21 -> [T55_4652_4632097164155]
  Demux/22 -> [T55_4653_4634320376545]

== system SSN_39busRT_Ctrl_4WT_19B/powergui/EquivalentModel11/Sources ==
  Mux : Mux  Inputs=[4 1 1 1 1 1 1 1]
  u : Outport  VectorParamsAs1DForOutWhenUnconnected=off
  wires:
  Mux/1 -> u/1
  [T175_15377_53253783684330] -> Mux/1
  [T160_13867_40125952328120] -> Mux/2
  [T160_13869_40179025857515] -> Mux/3
  [T161_13916_40005924062720] -> Mux/4
  [T161_13918_40059601977602] -> Mux/5
  [T75_6195_8148411547182] -> Mux/6
  [T75_6196_8149500738151] -> Mux/7
  [T75_6197_8150809302187] -> Mux/8

== system SSN_39busRT_Ctrl_4WT_19B/powergui/EquivalentModel11/Yout ==
  v,i : Inport
  Demux : Demux  Outputs=[4 1 1 1 1 1 1 1 1 1 1 1 1 1 1 1 1 1 1 1 1 1 1 1 1 1 1 1 1]
  tag scope: T124_10559_24030858426782=global, T124_10560_24038035941701=global, T124_10561_24045578783234=global, T124_10571_24168017419103=global, T124_10572_24175159908137=global, T124_10573_24182667723784=global, T160_13691_38888990411302=global, T160_13692_38898896230841=global, T160_13693_38909288641506=global, T160_13703_39078339118537=global, T160_13704_39088208698162=global, T160_13705_39098564868912=global, T166_14521_45417342626667=global, T166_14523_45465564786110=global, T167_14570_45399622716544=global, T167_14572_45448428622559=global, T175_15372_53078648363795=global, T176_15708_56967527514960=global, T177_15757_56782318453615=global, T177_15757_57115782414018=global, T177_15758_56783199454122=global, T177_15758_57113696116518=global, T178_15806_56932210227662=global, T178_15807_56930120730078=global, T178_15807_56933217384432=global, T178_15808_56931125143028=global, T78_6553_9763548218795=global, T78_6554_9764057438641=global, T78_6555_9764783684129=global
  wires:
  v,i/1 -> Demux/1
  Demux/1 -> [T175_15372_53078648363795]
  Demux/2 -> [T124_10571_24168017419103]
  Demux/3 -> [T124_10572_24175159908137]
  Demux/4 -> [T124_10573_24182667723784]
  Demux/5 -> [T160_13703_39078339118537]
  Demux/6 -> [T160_13704_39088208698162]
  Demux/7 -> [T160_13705_39098564868912]
  Demux/8 -> [T78_6553_9763548218795]
  Demux/9 -> [T78_6554_9764057438641]
  Demux/10 -> [T78_6555_9764783684129]
  Demux/11 -> [T124_10559_24030858426782]
  Demux/12 -> [T124_10560_24038035941701]
  Demux/13 -> [T124_10561_24045578783234]
  Demux/14 -> [T166_14521_45417342626667]
  Demux/15 -> [T166_14523_45465564786110]
  Demux/16 -> [T167_14570_45399622716544]
  Demux/17 -> [T167_14572_45448428622559]
  Demux/18 -> [T160_13691_38888990411302]
  Demux/19 -> [T160_13692_38898896230841]
  Demux/20 -> [T160_13693_38909288641506]
  Demux/21 -> [T176_15708_56967527514960]
  Demux/22 -> [T177_15757_56782318453615]
  Demux/23 -> [T177_15758_56783199454122]
  Demux/24 -> [T177_15757_57115782414018]
  Demux/25 -> [T178_15806_56932210227662]
  Demux/26 -> [T178_15807_56933217384432]
  Demux/27 -> [T177_15758_57113696116518]
  Demux/28 -> [T178_15807_56930120730078]
  Demux/29 -> [T178_15808_56931125143028]

== system SSN_39busRT_Ctrl_4WT_19B/powergui/EquivalentModel12/Sources ==
  Mux : Mux  Inputs=[4 1 1 1 1 1 1 1]
  u : Outport  VectorParamsAs1DForOutWhenUnconnected=off
  wires:
  Mux/1 -> u/1
  [T174_15332_52531863184100] -> Mux/1
  [T159_13822_39534117802891] -> Mux/2
  [T159_13824_39586699217718] -> Mux/3
  [T160_13871_39415689293204] -> Mux/4
  [T160_13873_39468875713961] -> Mux/5
  [T75_6197_8145913408919] -> Mux/6
  [T75_6198_8146998243020] -> Mux/7
  [T75_6199_8148302450187] -> Mux/8

== system SSN_39busRT_Ctrl_4WT_19B/powergui/EquivalentModel12/Yout ==
  v,i : Inport
  Demux : Demux  Outputs=[4 1 1 1 1 1 1 1 1 1 1 1 1 1 1 1 1 1 1 1 1 1 1 1 1 1 1 1 1]
  tag scope: T123_10514_23684299293976=global, T123_10515_23691324100464=global, T123_10516_23698710868578=global, T123_10526_23819103838046=global, T123_10527_23826093662175=global, T123_10528_23833445447930=global, T159_13646_38320859394156=global, T159_13647_38330629665695=global, T159_13648_38340883157359=global, T159_13658_38508049124770=global, T159_13659_38517783182886=global, T159_13660_38528000461128=global, T165_14476_44770942609293=global, T165_14478_44818685159776=global, T166_14525_44754801792774=global, T166_14527_44803128466565=global, T174_15327_52358042909016=global, T175_15663_56203939925085=global, T176_15712_56020882417453=global, T176_15712_56353703484071=global, T176_15713_56021688608452=global, T176_15713_56351553402270=global, T177_15761_56172256033349=global, T177_15762_56170103473718=global, T177_15762_56173188553194=global, T177_15763_56171033253233=global, T78_6555_9760124096012=global, T78_6556_9760629232076=global, T78_6557_9761351393781=global
  wires:
  v,i/1 -> Demux/1
  Demux/1 -> [T174_15327_52358042909016]
  Demux/2 -> [T123_10526_23819103838046]
  Demux/3 -> [T123_10527_23826093662175]
  Demux/4 -> [T123_10528_23833445447930]
  Demux/5 -> [T159_13658_38508049124770]
  Demux/6 -> [T159_13659_38517783182886]
  Demux/7 -> [T159_13660_38528000461128]
  Demux/8 -> [T78_6555_9760124096012]
  Demux/9 -> [T78_6556_9760629232076]
  Demux/10 -> [T78_6557_9761351393781]
  Demux/11 -> [T123_10514_23684299293976]
  Demux/12 -> [T123_10515_23691324100464]
  Demux/13 -> [T123_10516_23698710868578]
  Demux/14 -> [T165_14476_44770942609293]
  Demux/15 -> [T165_14478_44818685159776]
  Demux/16 -> [T166_14525_44754801792774]
  Demux/17 -> [T166_14527_44803128466565]
  Demux/18 -> [T159_13646_38320859394156]
  Demux/19 -> [T159_13647_38330629665695]
  Demux/20 -> [T159_13648_38340883157359]
  Demux/21 -> [T175_15663_56203939925085]
  Demux/22 -> [T176_15712_56020882417453]
  Demux/23 -> [T176_15713_56021688608452]
  Demux/24 -> [T176_15712_56353703484071]
  Demux/25 -> [T177_15761_56172256033349]
  Demux/26 -> [T177_15762_56173188553194]
  Demux/27 -> [T176_15713_56351553402270]
  Demux/28 -> [T177_15762_56170103473718]
  Demux/29 -> [T177_15763_56171033253233]

== system SSN_39busRT_Ctrl_4WT_19B/powergui/EquivalentModel13/Sources ==
  Mux : Mux  Inputs=[4 1 1 1 1 1 1 1]
  u : Outport  VectorParamsAs1DForOutWhenUnconnected=off
  wires:
  Mux/1 -> u/1
  [T175_15382_53226366560951] -> Mux/1
  [T160_13872_40101070870314] -> Mux/2
  [T160_13874_40154132477075] -> Mux/3
  [T161_13921_39981152564397] -> Mux/4
  [T161_13923_40034818628428] -> Mux/5
  [T75_6198_8144170888335] -> Mux/6
  [T75_6199_8145253820187] -> Mux/7
  [T75_6200_8146556125106] -> Mux/8

== system SSN_39busRT_Ctrl_4WT_19B/powergui/EquivalentModel13/Yout ==
  v,i : Inport
  Demux : Demux  Outputs=[4 1 1 1 1 1 1 1 1 1 1 1 1 1 1 1 1 1 1 1 1 1 1 1 1 1 1 1 1]
  tag scope: T124_10564_24012279052454=global, T124_10565_24019449105526=global, T124_10566_24026984485210=global, T124_10576_24149350049512=global, T124_10577_24156485076698=global, T124_10578_24163985430498=global, T160_13696_38865074330187=global, T160_13697_38874974285015=global, T160_13698_38885360830969=global, T160_13708_39054353588300=global, T160_13709_39064217303213=global, T160_13710_39074567609252=global, T166_14526_45391055690349=global, T166_14528_45439266811867=global, T167_14575_45373442368184=global, T167_14577_45422237297543=global, T175_15377_53051259387447=global, T176_15713_56938733071088=global, T177_15762_56753659401368=global, T177_15762_57087091931116=global, T177_15763_56754535044488=global, T177_15763_57085000907366=global, T178_15811_56903652745987=global, T178_15812_56901558575257=global, T178_15812_56904654574363=global, T178_15813_56902557659812=global, T78_6556_9758002751557=global, T78_6557_9758506104604=global, T78_6558_9759226483292=global
  wires:
  v,i/1 -> Demux/1
  Demux/1 -> [T175_15377_53051259387447]
  Demux/2 -> [T124_10576_24149350049512]
  Demux/3 -> [T124_10577_24156485076698]
  Demux/4 -> [T124_10578_24163985430498]
  Demux/5 -> [T160_13708_39054353588300]
  Demux/6 -> [T160_13709_39064217303213]
  Demux/7 -> [T160_13710_39074567609252]
  Demux/8 -> [T78_6556_9758002751557]
  Demux/9 -> [T78_6557_9758506104604]
  Demux/10 -> [T78_6558_9759226483292]
  Demux/11 -> [T124_10564_24012279052454]
  Demux/12 -> [T124_10565_24019449105526]
  Demux/13 -> [T124_10566_24026984485210]
  Demux/14 -> [T166_14526_45391055690349]
  Demux/15 -> [T166_14528_45439266811867]
  Demux/16 -> [T167_14575_45373442368184]
  Demux/17 -> [T167_14577_45422237297543]
  Demux/18 -> [T160_13696_38865074330187]
  Demux/19 -> [T160_13697_38874974285015]
  Demux/20 -> [T160_13698_38885360830969]
  Demux/21 -> [T176_15713_56938733071088]
  Demux/22 -> [T177_15762_56753659401368]
  Demux/23 -> [T177_15763_56754535044488]
  Demux/24 -> [T177_15762_57087091931116]
  Demux/25 -> [T178_15811_56903652745987]
  Demux/26 -> [T178_15812_56904654574363]
  Demux/27 -> [T177_15763_57085000907366]
  Demux/28 -> [T178_15812_56901558575257]
  Demux/29 -> [T178_15813_56902557659812]

== system SSN_39busRT_Ctrl_4WT_19B/powergui/EquivalentModel14/Sources ==
  Mux : Mux  Inputs=[1 1 1 1 1 1 1 1 1]
  u : Outport  VectorParamsAs1DForOutWhenUnconnected=off
  wires:
  Mux/1 -> u/1
  [T76_6244_8362903076491] -> Mux/1
  [T76_6245_8364077564632] -> Mux/2
  [T76_6246_8365474789614] -> Mux/3
  [T76_6247_8358771752988] -> Mux/4
  [T76_6248_8359940227233] -> Mux/5
  [T76_6249_8361331438321] -> Mux/6
  [T75_6197_8147012304955] -> Mux/7
  [T75_6198_8148096714155] -> Mux/8
  [T75_6199_8149400496422] -> Mux/9

== system SSN_39busRT_Ctrl_4WT_19B/powergui/EquivalentModel14/Yout ==
  v,i : Inport
  Demux : Demux  Outputs=[1 1 1 1 1 1 1 1 1 1 1 1]
  tag scope: T56_4731_4740275481815=global, T56_4732_4742115228519=global, T56_4733_4744525065494=global, T78_6555_9761080392463=global, T78_6556_9761585130258=global, T78_6557_9762306893695=global, T79_6602_10015198509971=global, T79_6603_10015788198676=global, T79_6604_10016598264343=global, T79_6605_10009809457747=global, T79_6606_10010393504846=global, T79_6607_10011197928906=global
  wires:
  v,i/1 -> Demux/1
  Demux/1 -> [T56_4731_4740275481815]
  Demux/2 -> [T56_4733_4744525065494]
  Demux/3 -> [T56_4732_4742115228519]
  Demux/4 -> [T79_6602_10015198509971]
  Demux/5 -> [T79_6603_10015788198676]
  Demux/6 -> [T79_6604_10016598264343]
  Demux/7 -> [T79_6605_10009809457747]
  Demux/8 -> [T79_6606_10010393504846]
  Demux/9 -> [T79_6607_10011197928906]
  Demux/10 -> [T78_6555_9761080392463]
  Demux/11 -> [T78_6556_9761585130258]
  Demux/12 -> [T78_6557_9762306893695]

== system SSN_39busRT_Ctrl_4WT_19B/powergui/EquivalentModel15/Sources ==
  Mux : Mux  Inputs=[1 1 1 1 1 1]
  u : Outport  VectorParamsAs1DForOutWhenUnconnected=off
  wires:
  Mux/1 -> u/1
  [T74_6156_7922838437025] -> Mux/1
  [T74_6157_7923822452664] -> Mux/2
  [T74_6158_7925022478032] -> Mux/3
  [T75_6209_8127005581668] -> Mux/4
  [T75_6210_8128068820998] -> Mux/5
  [T75_6211_8129351433395] -> Mux/6

== system SSN_39busRT_Ctrl_4WT_19B/powergui/EquivalentModel15/Yout ==
  v,i : Inport
  Demux : Demux  Outputs=[1 1 1 1 1 1 1 1 1]
  tag scope: T55_4687_4610159491098=global, T55_4688_4611848567960=global, T55_4689_4614102284916=global, T77_6514_9496751303322=global, T77_6515_9497161561183=global, T77_6516_9497785494108=global, T78_6567_9736884383576=global, T78_6568_9737369278415=global, T78_6569_9738071198894=global
  wires:
  v,i/1 -> Demux/1
  Demux/1 -> [T55_4687_4610159491098]
  Demux/2 -> [T55_4689_4614102284916]
  Demux/3 -> [T55_4688_4611848567960]
  Demux/4 -> [T77_6514_9496751303322]
  Demux/5 -> [T77_6515_9497161561183]
  Demux/6 -> [T77_6516_9497785494108]
  Demux/7 -> [T78_6567_9736884383576]
  Demux/8 -> [T78_6568_9737369278415]
  Demux/9 -> [T78_6569_9738071198894]

== system SSN_39busRT_Ctrl_4WT_19B/powergui/EquivalentModel16/Gates ==
  Mux : Mux  Inputs=[1 1 1]
  gates : Outport  VectorParamsAs1DForOutWhenUnconnected=off
  wires:
  Mux/1 -> gates/1
  [T69_6107_7468201614020] -> Mux/1
  [T69_6108_7471570481321] -> Mux/2
  [T69_6109_7475138548913] -> Mux/3

== system SSN_39busRT_Ctrl_4WT_19B/powergui/EquivalentModel16/Sources ==
  Mux : Mux  Inputs=[1 1 1 1 1 1]
  Mux_u : Mux  Inputs=[3 6]
  SwitchCurrents : Constant  Value=zeros(3,1)
  u : Outport  VectorParamsAs1DForOutWhenUnconnected=off
  wires:
  Mux_u/1 -> u/1
  SwitchCurrents/1 -> Mux_u/1
  Mux/1 -> Mux_u/2
  [T77_6303_8558738003612] -> Mux/1
  [T77_6304_8559981747457] -> Mux/2
  [T77_6305_8561451592341] -> Mux/3
  [T77_6304_8556974841015] -> Mux/4
  [T77_6305_8558216646159] -> Mux/5
  [T77_6306_8559684552341] -> Mux/6

== system SSN_39busRT_Ctrl_4WT_19B/powergui/EquivalentModel16/Status ==
  status : Inport
  Demux : Demux  Outputs=[1 1 1]
  tag scope: T71_6342_8413278393070=global, T71_6343_8416106367276=global, T71_6344_8419127930495=global
  wires:
  status/1 -> Demux/1
  Demux/1 -> [T71_6342_8413278393070]
  Demux/2 -> [T71_6343_8416106367276]
  Demux/3 -> [T71_6344_8419127930495]
